simulink model "sampleModel1615"  (R2023a)
settings: Solver=VariableStepAuto  StartTime=0.0  StopTime=10.0  RelTol=1e-3
libraries: hdlsllib x3, simulink x1
settings Model: Creator=user1  LastModifiedBy=user1

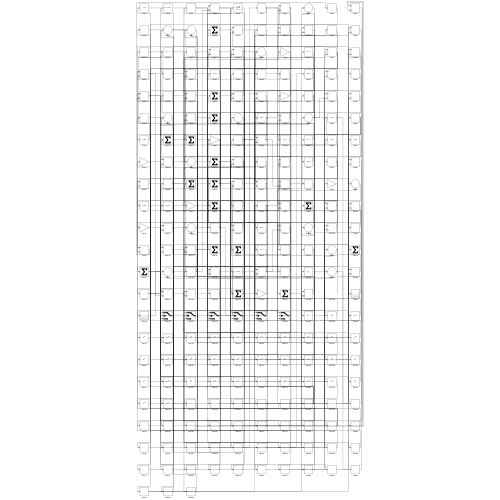
[thumbnail: Simulink's stored preview of the top-level diagram]
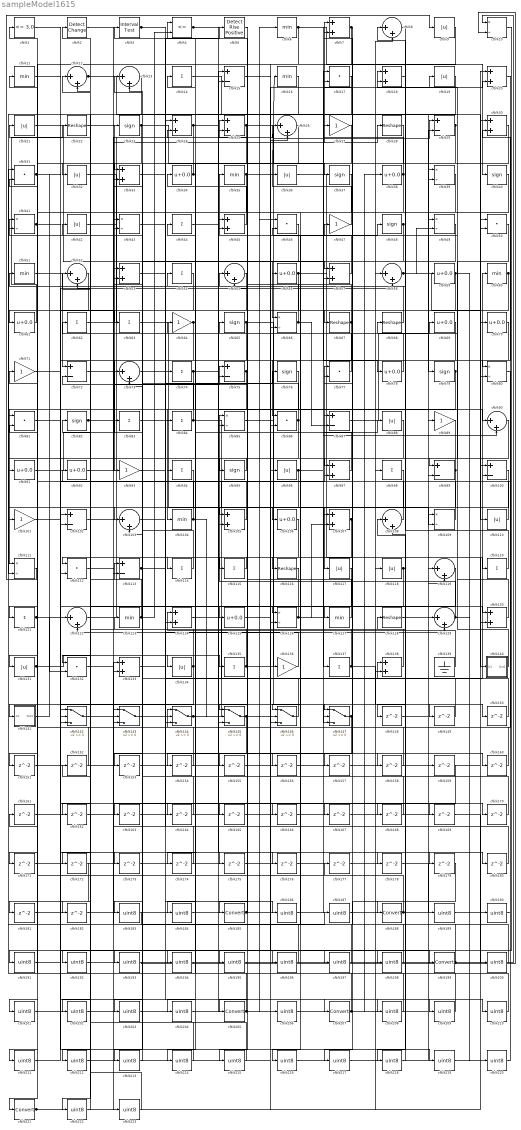
== system sampleModel1615 ==
  cfblk1 : hdlsllib/Logic and Bit Operations/Compare To Constant  relop=<=  const=3.0  OutDataTypeStr=boolean
  cfblk{10,39,41,43,49,66,80,85,109,111,126} (11 alike) : Product  Inputs=*/  RndMeth=Zero  SaturateOnIntegerOverflow=on
  cfblk{15,29,72,75,87,99..100,102,113} (9 alike) : Sum  Inputs=+-
  cfblk{27,47,64,71,89,93,101,136} (8 alike) : Gain
  cfblk{8,12..13,26,52,55,58,73,90,103,108,119,122,129} (14 alike) : Sum  Inputs=|++
  cfblk{6,11,16,35,51,60,104,123,127} (9 alike) : MinMax
  cfblk{7,18,20,24..25,30,33,45,53,57,97,105,107,124,130,133,138} (17 alike) : Sum
  cfblk{34,38,56,59,61,69..70,78,91..92,106,125} (12 alike) : Bias  Bias=0.0  SaturateOnIntegerOverflow=off
  cfblk{9,19,21,32,36,42,88,96,110,117..118,131,134} (13 alike) : Abs  SaturateOnIntegerOverflow=off
  cfblk{17,31,46,50,77,81,86,112,132} (9 alike) : DotProduct  OutDataTypeStr=Inherit: Inherit via internal rule
  cfblk{14,44,54,62..63,74,83..84,94,98,114..115,120..121,135,137} (16 alike) : Sum  Inputs=+
  cfblk{22,28,67..68,116,128} (6 alike) : Reshape
  cfblk139 : Ground
  cfblk140 : Subsystem
      settings: LibrarySourceBlock=|
      | hdlsllib/Ports &
      | Subsystems/Subsystem
  cfblk141 : Subsystem
      settings: LibrarySourceBlock=|
      | hdlsllib/Ports &
      | Subsystems/Subsystem
  cfblk{142..147} (6 alike) : Switch  SaturateOnIntegerOverflow=off  InputSameDT=off
  cfblk{148..182} (35 alike) : Delay  SampleTime=1
  cfblk{183..184,186..187,189..198,200..204,206,208..220,222..223} (35 alike) : DataTypeConversion  OutDataTypeStr=uint8  SaturateOnIntegerOverflow=off  RndMeth=Floor
  cfblk{185,188,199,205,207,221} (6 alike) : DataTypeConversion  SaturateOnIntegerOverflow=off  RndMeth=Floor
  cfblk2 : simulink/Logic and Bit Operations/Detect Change  vinit=0  OutDataTypeStr=boolean
      settings: LibrarySourceBlock=|
      | hdlsllib/Logic and Bit
      | Operations/Detect
      | Change
  cfblk{23,37,40,48,65,76,79,82,95} (9 alike) : Signum
  cfblk3 : hdlsllib/Logic and Bit Operations/Interval Test  IntervalClosedRight=on  uplimit=0.5  IntervalClosedLeft=on  lowlimit=-0.5  OutDataTypeStr=boolean
  cfblk4 : RelationalOperator  Operator=<=  OutDataTypeStr=boolean  InputSameDT=off
  cfblk5 : hdlsllib/Logic and Bit Operations/Detect Rise Positive  vinit=0  OutDataTypeStr=boolean
  wires:
  cfblk135/1 -> cfblk29/1, cfblk33/2
  cfblk68/1 -> cfblk54/1
  cfblk85/1 -> cfblk48/1
  cfblk59/1 -> cfblk18/1, cfblk151/1, cfblk190/1
  cfblk124/1 -> cfblk60/1
  cfblk67/1 -> cfblk25/1, cfblk145/3
  cfblk6/1 -> cfblk40/1, cfblk78/1, cfblk146/3
  cfblk129/1 -> cfblk85/1, cfblk220/1
  cfblk75/1 -> cfblk104/1, cfblk72/2
  cfblk45/1 -> cfblk34/1
  cfblk36/1 -> cfblk120/1
  cfblk63/1 -> cfblk117/1
  cfblk98/1 -> cfblk205/1
  cfblk35/1 -> cfblk16/1, cfblk131/1
  cfblk38/1 -> cfblk7/1, cfblk132/1, cfblk184/1
  cfblk139/1 -> cfblk124/1
  cfblk74/1 -> cfblk111/1, cfblk147/2, cfblk90/1
  cfblk20/1 -> cfblk80/1
  cfblk32/1 -> cfblk127/1
  cfblk111/1 -> cfblk9/1
  cfblk69/1 -> cfblk93/1
  cfblk87/1 -> cfblk69/1
  cfblk83/1 -> cfblk137/1
  cfblk91/1 -> cfblk23/1
  cfblk52/1 -> cfblk221/1
  cfblk108/1 -> cfblk92/1
  cfblk46/1 -> cfblk66/1
  cfblk19/1 -> cfblk111/2
  cfblk141/1(Out1) -> cfblk122/1
  cfblk110/1 -> cfblk18/2
  cfblk4/1 -> cfblk169/1, cfblk170/1
  cfblk137/1 -> cfblk73/2, cfblk149/1
  cfblk51/1 -> cfblk72/1
  cfblk99/1 -> cfblk121/1, cfblk97/1
  cfblk86/1 -> cfblk4/1, cfblk171/1, cfblk172/1
  cfblk65/1 -> cfblk147/1, cfblk20/2, cfblk163/1
  cfblk130/1 -> cfblk68/1
  cfblk34/1 -> cfblk84/1, cfblk33/1
  cfblk84/1 -> cfblk109/2, cfblk27/1, cfblk41/1
  cfblk21/1 -> cfblk57/1
  cfblk47/1 -> cfblk36/1
  cfblk56/1 -> cfblk140/1(In1), cfblk214/1
  cfblk109/1 -> cfblk83/1
  cfblk12/1 -> cfblk79/1, cfblk147/3
  cfblk62/1 -> cfblk25/2
  cfblk61/1 -> cfblk22/1
  cfblk44/1 -> cfblk35/1
  cfblk106/1 -> cfblk133/2
  cfblk104/1 -> cfblk2/1, cfblk145/2
  cfblk95/1 -> cfblk91/1
  cfblk80/1 -> cfblk144/1
  cfblk146/1 -> cfblk113/1
  cfblk131/1 -> cfblk134/1, cfblk97/2, cfblk166/1
  cfblk120/1 -> cfblk53/1
  cfblk58/1 -> cfblk110/1, cfblk8/1, cfblk49/2
  cfblk1/1 -> cfblk63/1
  cfblk27/1 -> cfblk94/1
  cfblk82/1 -> cfblk28/1, cfblk210/1
  cfblk79/1 -> cfblk153/1, cfblk201/1
  cfblk66/1 -> cfblk3/1, cfblk87/2
  cfblk60/1 -> cfblk86/2, cfblk105/2, cfblk168/1
  cfblk41/1 -> cfblk130/1, cfblk176/1
  cfblk92/1 -> cfblk75/1
  cfblk14/1 -> cfblk70/1
  cfblk143/1 -> cfblk138/1
  cfblk26/1 -> cfblk101/1
  cfblk29/1 -> cfblk114/1, cfblk145/1, cfblk126/2
  cfblk2/1 -> cfblk43/1
  cfblk123/1 -> cfblk42/1, cfblk4/2
  cfblk78/1 -> cfblk44/1
  cfblk126/1 -> cfblk88/1, cfblk125/1, cfblk107/2
  cfblk42/1 -> cfblk74/1
  cfblk70/1 -> cfblk86/1
  cfblk100/1 -> cfblk188/1
  cfblk24/1 -> cfblk32/1, cfblk179/1
  cfblk147/1 -> cfblk87/1, cfblk154/1
  cfblk55/1 -> cfblk103/1
  cfblk122/1 -> cfblk126/1
  cfblk114/1 -> cfblk51/1
  cfblk49/1 -> cfblk95/1
  cfblk144/1 -> cfblk77/1, cfblk146/2
  cfblk96/1 -> cfblk142/3, cfblk105/1, cfblk90/2, cfblk216/1
  cfblk15/1 -> cfblk199/1
  cfblk25/1 -> cfblk37/1, cfblk162/1
  cfblk23/1 -> cfblk136/1, cfblk181/1
  cfblk37/1 -> cfblk146/1
  cfblk31/1 -> cfblk132/2, cfblk178/1
  cfblk50/1 -> cfblk99/1
  cfblk9/1 -> cfblk144/2
  cfblk40/1 -> cfblk67/1
  cfblk116/1 -> cfblk124/2
  cfblk8/1 -> cfblk108/2
  cfblk142/1 -> cfblk143/2
  cfblk28/1 -> cfblk73/1
  cfblk121/1 -> cfblk58/2, cfblk144/3, cfblk193/1
  cfblk127/1 -> cfblk55/1
  cfblk64/1 -> cfblk142/2, cfblk204/1
  cfblk88/1 -> cfblk106/1
  cfblk77/1 -> cfblk62/1
  cfblk43/1 -> cfblk129/2
  cfblk140/1(Out1) -> cfblk45/1
  cfblk57/1 -> cfblk47/1
  cfblk3/1 -> cfblk175/1, cfblk186/1
  cfblk138/1 -> cfblk21/1
  cfblk7/1 -> cfblk61/1, cfblk157/1
  cfblk105/1 -> cfblk71/1
  cfblk93/1 -> cfblk5/1
  cfblk53/1 -> cfblk135/1
  cfblk54/1 -> cfblk113/2
  cfblk113/1 -> cfblk76/1, cfblk208/1
  cfblk115/1 -> cfblk112/1
  cfblk97/1 -> cfblk14/1
  cfblk103/1 -> cfblk26/1
  cfblk128/1 -> cfblk59/1
  cfblk136/1 -> cfblk122/2
  cfblk145/1 -> cfblk19/1, cfblk164/1
  cfblk118/1 -> cfblk182/1, cfblk198/1
  cfblk48/1 -> cfblk56/1, cfblk203/1
  cfblk107/1 -> cfblk116/1, cfblk115/1
  cfblk11/1 -> cfblk207/1
  cfblk17/1 -> cfblk185/1
  cfblk72/1 -> cfblk24/2
  cfblk134/1 -> cfblk141/1(In1), cfblk123/1
  cfblk18/1 -> cfblk148/1
  cfblk148/1 -> cfblk99/2
  cfblk149/1 -> cfblk109/1
  cfblk73/1 -> cfblk150/1
  cfblk150/1 -> cfblk75/2
  cfblk151/1 -> cfblk50/2
  cfblk152/1 -> cfblk142/1
  cfblk153/1 -> cfblk85/2
  cfblk154/1 -> cfblk1/1
  cfblk5/1 -> cfblk155/1
  cfblk155/1 -> cfblk66/2
  cfblk133/1 -> cfblk156/1
  cfblk156/1 -> cfblk20/1
  cfblk157/1 -> cfblk77/2
  cfblk22/1 -> cfblk158/1
  cfblk158/1 -> cfblk55/2
  cfblk132/1 -> cfblk160/1
  cfblk160/1 -> cfblk108/1
  cfblk161/1 -> cfblk80/2
  cfblk163/1 -> cfblk103/2
  cfblk164/1 -> cfblk43/2
  cfblk16/1 -> cfblk165/1
  cfblk165/1 -> cfblk129/1
  cfblk166/1 -> cfblk57/2
  cfblk125/1 -> cfblk167/1
  cfblk167/1 -> cfblk58/1
  cfblk168/1 -> cfblk53/2
  cfblk170/1 -> cfblk45/2
  cfblk171/1 -> cfblk143/3
  cfblk71/1 -> cfblk173/1
  cfblk173/1 -> cfblk107/1
  cfblk90/1 -> cfblk174/1
  cfblk174/1 -> cfblk24/1
  cfblk175/1 -> cfblk26/2
  cfblk176/1 -> cfblk29/2
  cfblk177/1 -> cfblk8/2
  cfblk33/1 -> cfblk180/1
  cfblk180/1 -> cfblk143/1
  cfblk181/1 -> cfblk49/1
  cfblk159/1 -> cfblk183/1
  cfblk184/1 -> cfblk159/1
  cfblk185/1 -> cfblk130/2, cfblk6/1, cfblk65/1
  cfblk186/1 -> cfblk17/1
  cfblk183/1 -> cfblk187/1
  cfblk187/1 -> cfblk17/2
  cfblk188/1 -> cfblk177/1, cfblk152/1, cfblk31/2, cfblk12/2
  cfblk178/1 -> cfblk189/1
  cfblk189/1 -> cfblk100/1
  cfblk190/1 -> cfblk100/2
  cfblk10/1 -> cfblk191/1
  cfblk191/1 -> cfblk112/2
  cfblk76/1 -> cfblk192/1
  cfblk192/1 -> cfblk10/1
  cfblk193/1 -> cfblk10/2
  cfblk89/1 -> cfblk194/1
  cfblk194/1 -> cfblk118/1
  cfblk182/1 -> cfblk195/1
  cfblk195/1 -> cfblk89/1
  cfblk81/1 -> cfblk196/1
  cfblk196/1 -> cfblk133/1
  cfblk112/1 -> cfblk197/1
  cfblk197/1 -> cfblk81/1
  cfblk198/1 -> cfblk81/2
  cfblk199/1 -> cfblk41/2, cfblk7/2, cfblk46/2
  cfblk169/1 -> cfblk200/1
  cfblk200/1 -> cfblk15/1
  cfblk201/1 -> cfblk15/2
  cfblk119/1 -> cfblk202/1
  cfblk202/1 -> cfblk12/1
  cfblk203/1 -> cfblk119/1
  cfblk204/1 -> cfblk119/2
  cfblk205/1 -> cfblk31/1, cfblk46/1
  cfblk206/1 -> cfblk98/1
  cfblk207/1 -> cfblk161/1, cfblk38/1
  cfblk208/1 -> cfblk11/1
  cfblk102/1 -> cfblk209/1
  cfblk209/1 -> cfblk64/1
  cfblk210/1 -> cfblk102/1
  cfblk172/1 -> cfblk211/1
  cfblk211/1 -> cfblk102/2
  cfblk13/1 -> cfblk212/1
  cfblk212/1 -> cfblk96/1
  cfblk94/1 -> cfblk213/1
  cfblk213/1 -> cfblk13/1
  cfblk214/1 -> cfblk13/2
  cfblk39/1 -> cfblk215/1
  cfblk215/1 -> cfblk82/1
  cfblk216/1 -> cfblk39/1
  cfblk179/1 -> cfblk217/1
  cfblk217/1 -> cfblk39/2
  cfblk30/1 -> cfblk218/1
  cfblk218/1 -> cfblk128/1
  cfblk101/1 -> cfblk219/1
  cfblk219/1 -> cfblk30/1
  cfblk220/1 -> cfblk30/2
  cfblk221/1 -> cfblk206/1, cfblk138/2, cfblk50/1
  cfblk117/1 -> cfblk222/1
  cfblk222/1 -> cfblk52/1
  cfblk162/1 -> cfblk223/1
  cfblk223/1 -> cfblk52/2

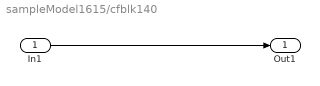
== system sampleModel1615/cfblk140 ==
  In1 : Inport
  Out1 : Outport
  wires:
  In1/1 -> Out1/1

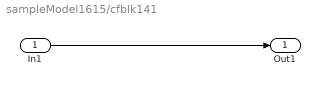
== system sampleModel1615/cfblk141 ==
  In1 : Inport
  Out1 : Outport
  wires:
  In1/1 -> Out1/1
